simulink model "simple_ode"  (R2020a)
settings: Solver=VariableStepAuto  StartTime=0.0  StopTime=10.0  RelTol=1e-3
settings Model: Creator=ch17d012  LastModifiedBy=ch17d012

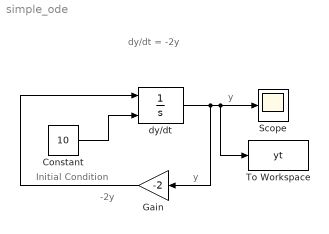
== system simple_ode ==
  note: dy/dt = -2y
  note: Initial Condition
  note: -2y
  note: y
  note: y
  Constant : Constant  Value=10
  Gain : Gain  Gain=-2
  Scope : Scope
  To Workspace : ToWorkspace  VariableName=yt  SaveFormat=Timeseries  SampleTime=-1
  dy/dt : Integrator  InitialConditionSource=external  InitialCondition=10
  wires:
  dy/dt/1 -> Gain/1, To Workspace/1, Scope/1
  Gain/1 -> dy/dt/1
  Constant/1 -> dy/dt/2
